simulink model "Arm_Simulation"  (R2022b)
settings: Solver=ode23t  StartTime=0.0  StopTime=10  RelTol=1e-3
undefined symbols (not defined in the file or in its folder): alpha, LF, Ts, X, Y, Z
libraries: sm_lib x16, nesl_utility x8, spsEdgeDetectorLib x6, instrumentseriallib x3, simulink_extras x3, simulink x2, svdutilitieslib x1
(part 1 of 2)
settings Model: PacingRate=10  Creator=gotta  LastModifiedBy=gotta
settings ExplorerConfigSet: InternalSimMechanicsExplorerSettings="<ExplorerConfiguration><canonicalview>default</canonicalview><AnimationSetting><BasePlaybackSpeed>1.0</BasePlaybackSpeed><PlaybackSpeedFactor>1.0</PlaybackSpeedFactor></AnimationSetting><TilePanel><TileInfo><Tiles Columns=\"2\" Count=\"3\" Rows=\"2\"><Column Weight=\"0.4994\"/><Column Weight=\"0.5006\"/><Row Weight=\"0.4993\"/><Row Weight=\"0.5007\"/><Tile Height=\"2\" Width=\"1\" X=\"0\" Y=\"0\"/><Tile Height=\"1\" Width=\"1\" X=\"1\" Y=\"0\"/><Tile Height=\"1\" Width=\"1\" X=\"1\" Y=\"1\"/></Tiles></TileInfo><SceneInfo><SceneViewer><BGColor><R>0.60000002384185791</R><G>0.60000002384185791</G><B>0.60000002384185791</B></BGColor><Camera><DoPerspective>off</DoPerspective><Position><X>0.130605904800483619</X><Y>-1.03965353021318974</Y><Z>0.165975841105155203</Z></Position><Center><X>0.130605904800483619</X><Y>-0.039653530213189736</Y><Z>0.165975841105155203</Z></Center><Up><X>0</X><Y>-0</Y><Z>1</Z></Up><ViewLimDist>1</ViewLimDist><YLim>0.285256663070233507</YLim><XLim>0.289401740076538072</XLim></Camera></SceneViewer><SceneViewer><BGColor><R>0.60000002384185791</R><G>0.60000002384185791</G><B>0.60000002384185791</B></BGColor><Camera><DoPerspective>off</DoPerspective><Position><X>0.102066420747171926</X><Y>-0.000570082663057591005</Y><Z>1.10062331896404597</Z></Position><Center><X>0.102066420747171926</X><Y>-0.000570082663057591005</Y><Z>0.100623318964045971</Z></Center><Up><X>0</X><Y>1</Y><Z>-0</Z></Up><ViewLimDist>1</ViewLimDist><YLim>0.171233923815175632</YLim><XLim>0.352540431384185116</XLim></Camera></SceneViewer><SceneViewer><BGColor><R>0.60000002384185791</R><G>0.60000002384185791</G><B>0.60000002384185791</B></BGColor><Camera><DoPerspective>off</DoPerspective><Position><X>1.08629246460336626</X><Y>-0.00159593778916227759</Y><Z>0.183546684797173593</Z></Position><Center><X>0.086292464603366259</X><Y>-0.00159593778916227759</Y><Z>0.183546684797173593</Z></Center><Up><X>-0</X><Y>0</Y><Z>1</Z></Up><ViewLimDist>1</ViewLimDist><YLim>0.219665879586588786</YLim><XLim>0.452253281501800386</XLim></Camera></SceneViewer></SceneInfo></TilePanel><MechEditorPanel><Cameras/><GfxPanelCameraMap/><VideoCreator><PlaybackSpeedRatio>1.0</PlaybackSpeedRatio><FrameRate>30</FrameRate><VideoFormat>Motion JPEG AVI</VideoFormat><FrameSize>auto</FrameSize></VideoCreator></MechEditorPanel></ExplorerConfiguration>"

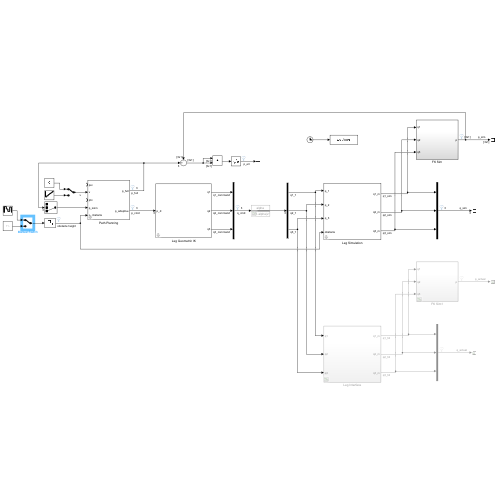
[thumbnail: Simulink's stored preview of the top-level diagram]
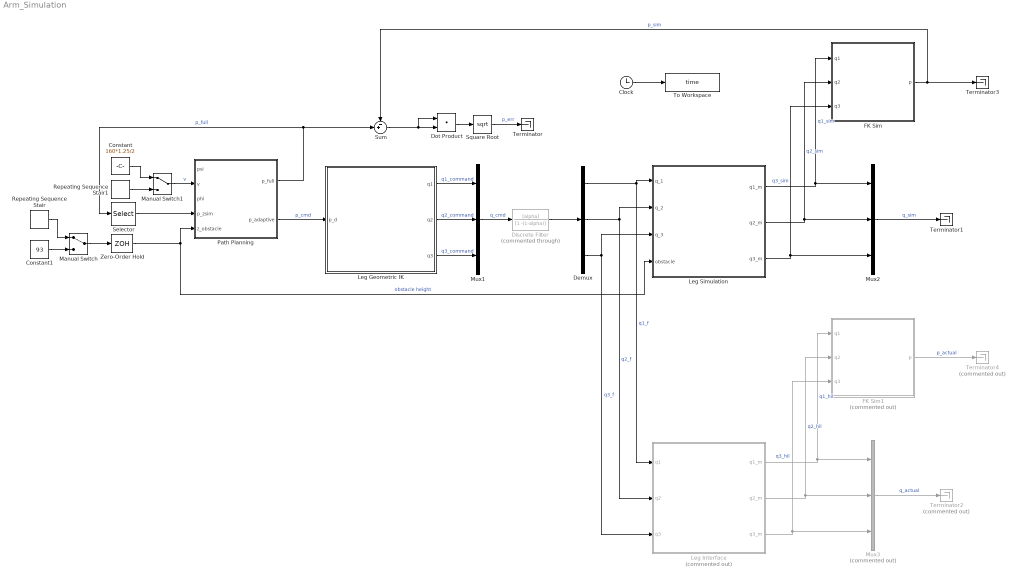
== system Arm_Simulation ==
  " Leg Geometric IK" : Subsystem  mask{coxa_length=40, femur_length=78, tibia_length=132, offset=178}
      mask prompts: coxa_length "Coxa Length [mm]:"; femur_length "Femur Length [mm]:"; tibia_length "Tibia Length [mm]:"; offset "Offset [mm]:"
  Clock : Clock
  Constant : Constant  Value=160*1.25/2
  Constant1 : Constant  Value=93
  Demux : Demux  Outputs=3
  Discrete Filter : DiscreteFilter  Commented=through  Numerator=[alpha]  Denominator=[1 -(1-alpha)]  SampleTime=Ts
  Dot Product : DotProduct  OutDataTypeStr=Inherit: Inherit via internal rule
  FK Sim : Subsystem
  FK Sim1 : Subsystem  Commented=on
  Leg Interface : Subsystem  Commented=on
  Leg Simulation : Subsystem  mask{RotationAngle=0.0}
      mask prompts: RotationAngle "Angular Offset [deg]:"
      mask TypeOptions RotationAngle: rotation/RotationAngle
  Manual Switch : ManualSwitch
  Manual Switch1 : ManualSwitch
  Mux1 : Mux  Inputs=3
  Mux2 : Mux  Inputs=3
  Mux3 : Mux  Commented=on  Inputs=3
  Path Planning : Subsystem  mask{Cx=155, Cy=0, Cz=93, r_o=60, n=1000, beta=0.6}
      mask prompts: Cx "X"; Cy "Y"; Cz "Z"; r_o "OWR Radius [mm]:"; n "Samples per Cycle:"; beta "Duty Factor beta:"
      mask DialogControl ParameterGroupVar Prompt: Rest Position [mm]
  Repeating Sequence Stair : simulink/Sources/Repeating Sequence Stair  OutValues=[93, 140, 140, 120, 120, 100, 100, 135, 135, 93]  tsamp=1  OutMin=[]  OutMax=[]  OutDataTypeStr=double  OutputDataTypeScalingMode=double  OutDataType=fixdt(0,8)  ConRadixGroup=Best Precision: Vector-wise  OutScaling=2^-12
  Repeating Sequence Stair1 : simulink/Sources/Repeating Sequence Stair  OutValues=[67:67/5:134]  tsamp=5  OutMin=[]  OutMax=[]  OutDataTypeStr=double  OutputDataTypeScalingMode=double  OutDataType=fixdt(0,8)  ConRadixGroup=Best Precision: Vector-wise  OutScaling=2^-12
  Selector : Selector  InputPortWidth=3  IndexOptions=Index vector (dialog)  Indices=3  OutputSizes=1
  Square Root : Sqrt
  Sum : Sum  Inputs=-+|
  Terminator : Terminator
  Terminator1 : Terminator
  Terminator2 : Terminator  Commented=on
  Terminator3 : Terminator
  Terminator4 : Terminator  Commented=on
  To Workspace : ToWorkspace  VariableName=time  SampleTime=1e-4
      settings: Save2DSignal=2-D array (concatenate along first dimension)
  Zero-Order Hold : ZeroOrderHold  SampleTime=1e-3
  wires:
  Leg Interface/3(q3_m) -> FK Sim1/3(q3), Mux3/3  "q3_hil"
  Leg Interface/2(q2_m) -> FK Sim1/2(q2), Mux3/2  "q2_hil"
  Leg Interface/1(q1_m) -> FK Sim1/1(q1), Mux3/1  "q1_hil"
  Leg Simulation/3(q3_m) -> Mux2/3, FK Sim/3(q3)  "q3_sim"
  Leg Simulation/2(q2_m) -> Mux2/2, FK Sim/2(q2)  "q2_sim"
  Leg Simulation/1(q1_m) -> Mux2/1, FK Sim/1(q1)  "q1_sim"
  Path Planning/1(p_full) -> Sum/2, Selector/1  "p_full"
  FK Sim/1(p) -> Terminator3/1, Sum/1  "p_sim"
  " Leg Geometric IK"/3(q3) -> Mux1/3  "q3_command"
  " Leg Geometric IK"/2(q2) -> Mux1/2  "q2_command"
  " Leg Geometric IK"/1(q1) -> Mux1/1  "q1_command"
  Demux/1 -> Leg Interface/1(q1), Leg Simulation/1(q_1)  "q1_f"
  Demux/2 -> Leg Interface/2(q2), Leg Simulation/2(q_2)  "q2_f"
  Demux/3 -> Leg Interface/3(q3), Leg Simulation/3(q_3)  "q3_f"
  Mux1/1 -> Discrete Filter/1  "q_cmd"
  Discrete Filter/1 -> Demux/1
  Constant/1 -> Manual Switch1/1
  Mux2/1 -> Terminator1/1  "q_sim"
  Mux3/1 -> Terminator2/1  "q_actual"
  FK Sim1/1(p) -> Terminator4/1  "p_actual"
  Selector/1 -> Path Planning/4(p_zsim)
  Repeating Sequence Stair1/1 -> Manual Switch1/2
  Manual Switch1/1 -> Path Planning/2(v)  "v"
  Clock/1 -> To Workspace/1
  Sum/1 -> Dot Product/1, Dot Product/2
  Dot Product/1 -> Square Root/1
  Square Root/1 -> Terminator/1  "p_err"
  Repeating Sequence Stair/1 -> Manual Switch/1
  Zero-Order Hold/1 -> Leg Simulation/4(obstacle), Path Planning/5(z_obstacle)  "obstacle height"
  Path Planning/2(p_adaptive) -> " Leg Geometric IK"/1(p_d)  "p_cmd"
  Constant1/1 -> Manual Switch/2
  Manual Switch/1 -> Zero-Order Hold/1

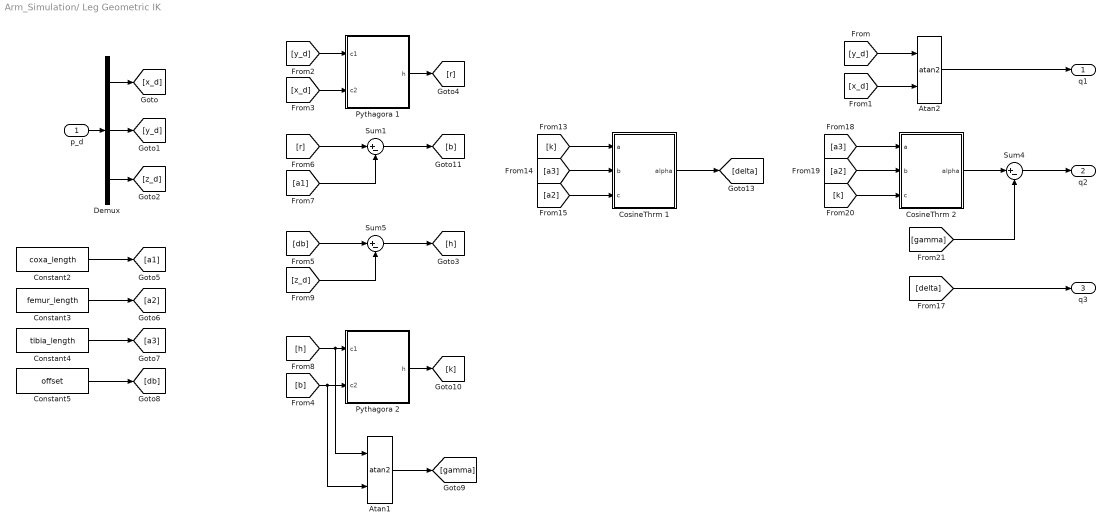
== system Arm_Simulation/ Leg Geometric IK ==
  p_d : Inport
  Atan1 : Trigonometry  Operator=atan2
  Atan2 : Trigonometry  Operator=atan2
  Constant2 : Constant  Value=coxa_length
  Constant3 : Constant  Value=femur_length
  Constant4 : Constant  Value=tibia_length
  Constant5 : Constant  Value=offset
  CosineThrm 1 : Subsystem
  CosineThrm 2 : Subsystem
  Demux : Demux  Outputs=3
  Pythagora 1 : Subsystem
  Pythagora 2 : Subsystem
  Sum1 : Sum  Inputs=|+-
  Sum4 : Sum  Inputs=|+-
  Sum5 : Sum  Inputs=|+-
  q1 : Outport
  q2 : Outport  Port=2
  q3 : Outport  Port=3
  wires:
  p_d/1 -> Demux/1
  Demux/3 -> [z_d]
  Atan2/1 -> q1/1
  Demux/1 -> [x_d]
  Demux/2 -> [y_d]
  [y_d] -> Atan2/1
  [x_d] -> Atan2/2
  Pythagora 1/1(h) -> [r]
  [y_d] -> Pythagora 1/1(c1)
  [x_d] -> Pythagora 1/2(c2)
  Constant4/1 -> [a3]
  Constant3/1 -> [a2]
  Constant2/1 -> [a1]
  [a1] -> Sum1/2
  [r] -> Sum1/1
  Sum1/1 -> [b]
  [b] -> Atan1/2, Pythagora 2/2(c2)
  [h] -> Atan1/1, Pythagora 2/1(c1)
  Pythagora 2/1(h) -> [k]
  CosineThrm 1/1(alpha) -> [delta]
  [a2] -> CosineThrm 1/3(c)
  [a3] -> CosineThrm 1/2(b)
  [k] -> CosineThrm 1/1(a)
  [a3] -> CosineThrm 2/1(a)
  [a2] -> CosineThrm 2/2(b)
  [k] -> CosineThrm 2/3(c)
  CosineThrm 2/1(alpha) -> Sum4/1
  Sum4/1 -> q2/1
  [gamma] -> Sum4/2
  Sum5/1 -> [h]
  [db] -> Sum5/1
  [z_d] -> Sum5/2
  Constant5/1 -> [db]
  Atan1/1 -> [gamma]
  [delta] -> q3/1

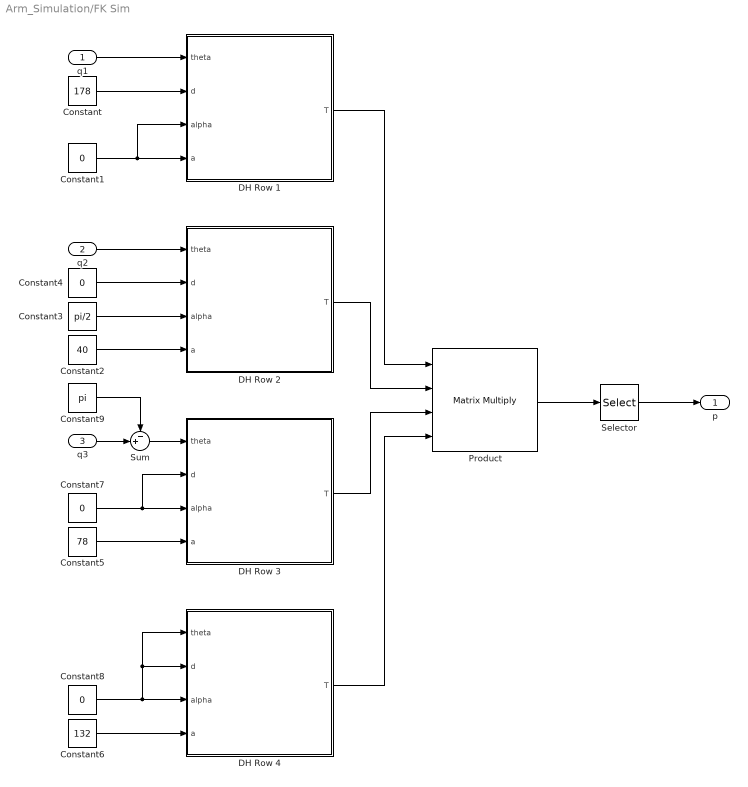
== system Arm_Simulation/FK Sim ==
  q1 : Inport
  q2 : Inport  Port=2
  q3 : Inport  Port=3
  Constant : Constant  Value=178
  Constant{1,4,7..8} (4 alike) : Constant  Value=0
  Constant2 : Constant  Value=40
  Constant3 : Constant  Value=pi/2
  Constant5 : Constant  Value=78
  Constant6 : Constant  Value=132
  Constant9 : Constant  Value=pi
  DH Row 1 : MATLAB Function  TreatAsAtomicUnit=on
  DH Row 2 : MATLAB Function  TreatAsAtomicUnit=on
  DH Row 3 : MATLAB Function  TreatAsAtomicUnit=on
  DH Row 4 : MATLAB Function  TreatAsAtomicUnit=on
  Product : Product  Inputs=4  Multiplication=Matrix(*)
  Selector : Selector  NumberOfDimensions=2  InputPortWidth=3  IndexOptions=Index vector (dialog),Index vector (dialog)  Indices=[1 2 3],4  OutputSizes=1,1
  Sum : Sum  Inputs=-+|
  p : Outport
  wires:
  q1/1 -> DH Row 1/1(theta)
  Constant/1 -> DH Row 1/2(d)
  Constant1/1 -> DH Row 1/3(alpha), DH Row 1/4(a)
  q2/1 -> DH Row 2/1(theta)
  Constant4/1 -> DH Row 2/2(d)
  Constant3/1 -> DH Row 2/3(alpha)
  Constant2/1 -> DH Row 2/4(a)
  Constant5/1 -> DH Row 3/4(a)
  Constant7/1 -> DH Row 3/3(alpha), DH Row 3/2(d)
  q3/1 -> Sum/2
  Constant8/1 -> DH Row 4/3(alpha), DH Row 4/1(theta), DH Row 4/2(d)
  Constant6/1 -> DH Row 4/4(a)
  DH Row 1/1(T) -> Product/1
  DH Row 2/1(T) -> Product/2
  DH Row 3/1(T) -> Product/3
  DH Row 4/1(T) -> Product/4
  Product/1 -> Selector/1
  Selector/1 -> p/1
  Sum/1 -> DH Row 3/1(theta)
  Constant9/1 -> Sum/1

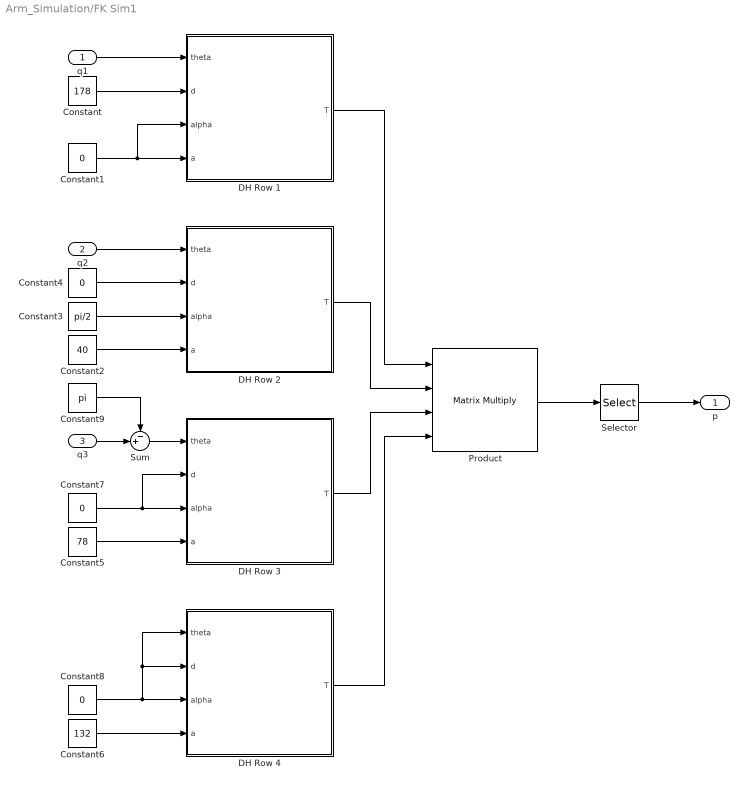
== system Arm_Simulation/FK Sim1 ==
  q1 : Inport
  q2 : Inport  Port=2
  q3 : Inport  Port=3
  Constant : Constant  Value=178
  Constant{1,4,7..8} (4 alike) : Constant  Value=0
  Constant2 : Constant  Value=40
  Constant3 : Constant  Value=pi/2
  Constant5 : Constant  Value=78
  Constant6 : Constant  Value=132
  Constant9 : Constant  Value=pi
  DH Row 1 : MATLAB Function  TreatAsAtomicUnit=on
  DH Row 2 : MATLAB Function  TreatAsAtomicUnit=on
  DH Row 3 : MATLAB Function  TreatAsAtomicUnit=on
  DH Row 4 : MATLAB Function  TreatAsAtomicUnit=on
  Product : Product  Inputs=4  Multiplication=Matrix(*)
  Selector : Selector  NumberOfDimensions=2  InputPortWidth=3  IndexOptions=Index vector (dialog),Index vector (dialog)  Indices=[1 2 3],4  OutputSizes=1,1
  Sum : Sum  Inputs=-+|
  p : Outport
  wires:
  Constant9/1 -> Sum/1
  Sum/1 -> DH Row 3/1(theta)
  Selector/1 -> p/1
  Product/1 -> Selector/1
  DH Row 4/1(T) -> Product/4
  DH Row 3/1(T) -> Product/3
  DH Row 2/1(T) -> Product/2
  DH Row 1/1(T) -> Product/1
  Constant6/1 -> DH Row 4/4(a)
  Constant8/1 -> DH Row 4/2(d), DH Row 4/1(theta), DH Row 4/3(alpha)
  q3/1 -> Sum/2
  Constant7/1 -> DH Row 3/2(d), DH Row 3/3(alpha)
  Constant5/1 -> DH Row 3/4(a)
  Constant2/1 -> DH Row 2/4(a)
  Constant3/1 -> DH Row 2/3(alpha)
  Constant4/1 -> DH Row 2/2(d)
  q2/1 -> DH Row 2/1(theta)
  Constant1/1 -> DH Row 1/4(a), DH Row 1/3(alpha)
  Constant/1 -> DH Row 1/2(d)
  q1/1 -> DH Row 1/1(theta)

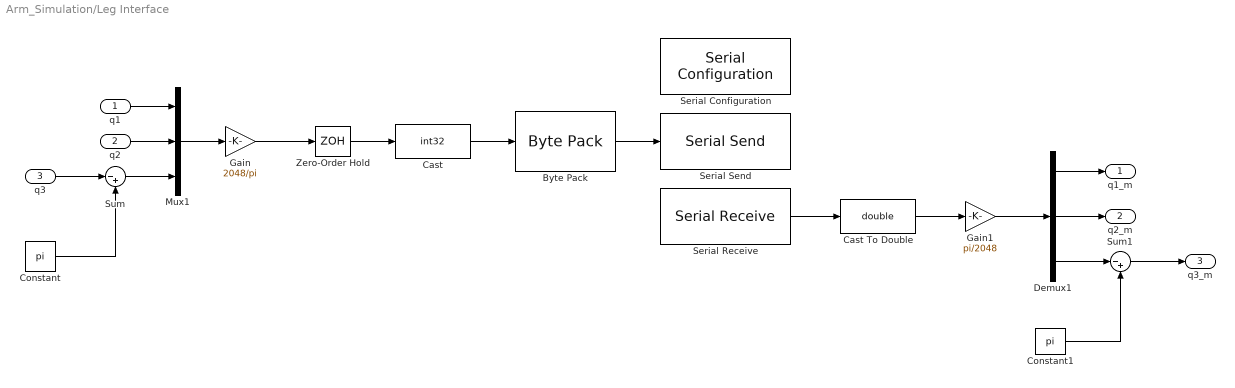
== system Arm_Simulation/Leg Interface ==
  q1 : Inport
  q2 : Inport  Port=2
  q3 : Inport  Port=3
  Byte Pack : svdutilitieslib/Byte Pack  maskPackedDataType=uint8  datatypes={'int32'}  byteAlign=1  blockPlatform=arduinoert
  Cast : DataTypeConversion  OutDataTypeStr=int32  SaturateOnIntegerOverflow=off  RndMeth=Floor
  Cast To Double : DataTypeConversion  OutDataTypeStr=double  SaturateOnIntegerOverflow=off  RndMeth=Floor
  Constant : Constant  Value=pi
  Constant1 : Constant  Value=pi
  Demux1 : Demux  Outputs=3
  Gain : Gain  Gain=2048/pi
  Gain1 : Gain  Gain=pi/2048
  Mux1 : Mux  Inputs=3
  Serial Configuration : instrumentseriallib/Serial Configuration  Priority=-200000  PortSel=COM6  Port=COM6  ComPort=COM6  BaudRate=115200  DataBits=8  Parity=none  StopBits=1  ByteOrder=little-endian  FlowControl=none  Timeout=10  SimulateUsing=Interpreted execution  BlockInModel=on  aMode=1
  Serial Receive : instrumentseriallib/Serial Receive  Priority=1  PortSel=COM6  Port=COM6  ComPort=COM6  DataType=int32  SaveDataType=uint8  ToggleHeader=on  Header='A'  ToggleTerminator=on  Terminator=LF ('\n')  CustomTerminator=[]  InputFormat=Column major  ToggleDataSize=on  DataSize=[1 3]  EnableBlockingMode=on  ActionDataUnavailable=Output last received value  ActionWhenDataUnavailable=Output last received value  CustomValue=0  SampleTime=1e-2  SimulateUsing=Interpreted execution  BlockInModel=on  aMode=1
  Serial Send : instrumentseriallib/Serial Send  Priority=1  PortSel=COM6  Port=COM6  ComPort=COM6  Header=[]  Terminator=<none>  CustomTerminator=[]  EnableBlockingMode=on  SimulateUsing=Interpreted execution  BlockInModel=on  aMode=1
  Sum : Sum  Inputs=|-+
  Sum1 : Sum  Inputs=|-+
  Zero-Order Hold : ZeroOrderHold  SampleTime=1e-2
  q1_m : Outport
  q2_m : Outport  Port=2
  q3_m : Outport  Port=3
  wires:
  Cast/1 -> Byte Pack/1
  Serial Receive/1 -> Cast To Double/1
  Mux1/1 -> Gain/1
  Demux1/2 -> q2_m/1
  Demux1/1 -> q1_m/1
  q1/1 -> Mux1/1
  q2/1 -> Mux1/2
  Cast To Double/1 -> Gain1/1
  Gain1/1 -> Demux1/1
  Gain/1 -> Zero-Order Hold/1
  Byte Pack/1 -> Serial Send/1
  Zero-Order Hold/1 -> Cast/1
  Sum/1 -> Mux1/3
  q3/1 -> Sum/1
  Constant/1 -> Sum/2
  Constant1/1 -> Sum1/2
  Sum1/1 -> q3_m/1
  Demux1/3 -> Sum1/1

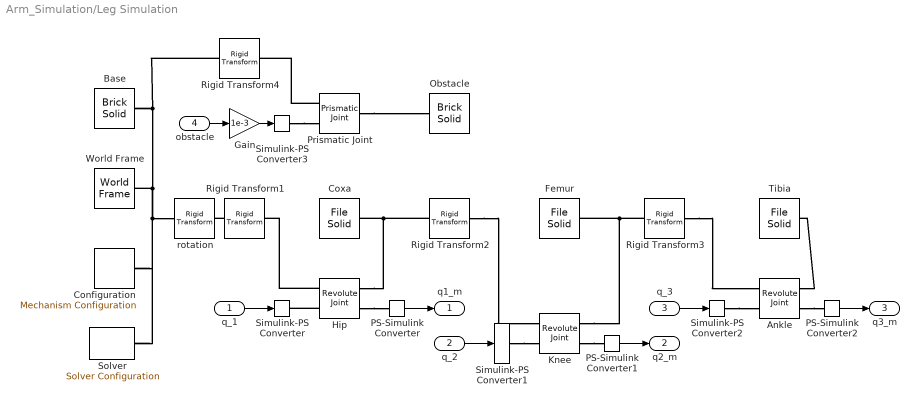
== system Arm_Simulation/Leg Simulation ==
  q_1 : Inport
  q_2 : Inport  Port=2
  q_3 : Inport  Port=3
  obstacle : Inport  Port=4
  Ankle : sm_lib/Joints/Revolute Joint  JointMode=Normal  SenseConstraintForce=off  SenseConstraintForceX=off  SenseConstraintForceY=off  SenseConstraintForceZ=off  SenseConstraintTorque=off  SenseConstraintTorqueX=off  SenseConstraintTorqueY=off  SenseConstraintTorqueZ=off  SenseTotalForce=off  SenseTotalForceX=off  SenseTotalForceY=off  SenseTotalForceZ=off  SenseTotalTorque=off  SenseTotalTorqueX=off  SenseTotalTorqueY=off  SenseTotalTorqueZ=off  CompositeWrenchDir=FollowerOnBase  CompositeWrenchFrame=BaseFrame  EquilibriumPosition=0  EquilibriumPositionUnits=deg  SpringStiffness=0  SpringStiffnessUnits=N*m/deg  DampingCoefficient=0  DampingCoefficientUnits=N*m/(deg/s)  TorqueActuationMode=ComputedTorque  MotionActuationMode=InputMotion  SensePosition=on  SenseVelocity=off  SenseAcceleration=off  SenseTorqueForce=off  SenseLowerLimitTorqueForce=off  SenseUpperLimitTorqueForce=off  LowerLimitSpecify=off  LowerLimitBound=-90  LowerLimitBoundUnits=deg  LowerLimitStiffness=1e4  LowerLimitStiffnessUnits=N*m/deg  LowerLimitDamping=10  LowerLimitDampingUnits=N*m/(deg/s)  LowerLimitTransitionRegionWidth=0.1  LowerLimitTransitionRegionWidthUnits=deg  UpperLimitSpecify=off  UpperLimitBound=90  UpperLimitBoundUnits=deg  UpperLimitStiffness=1e4  UpperLimitStiffnessUnits=N*m/deg  UpperLimitDamping=10  UpperLimitDampingUnits=N*m/(deg/s)  UpperLimitTransitionRegionWidth=0.1  UpperLimitTransitionRegionWidthUnits=deg  PositionTargetSpecify=off  PositionTargetPriority=High  PositionTargetValue=0  PositionTargetValueUnits=deg  VelocityTargetSpecify=off  VelocityTargetPriority=High  VelocityTargetValue=0  VelocityTargetValueUnits=deg/s
  Base : sm_lib/Body Elements/Brick Solid  GraphicAmbientColor=[0.15 0.15 0.15 1.0]  BasedOnType=Density  BrickDimensions=[15 15 200]  BrickDimensionUnits=mm  CenterOfMass=[0 0 0]  CenterOfMassUnits=m  GraphicDiffuseColor=[0.0 0.0 0.0]  Density=1000  DensityUnits=kg/m^3  DoExposeReferenceFrame=on  GraphicEmissiveColor=[0.0 0.0 0.0 1.0]  ExportEntireGeometry=off  SerializedFrames=<Frames><Frame><Id>Frame1</Id><Value><Name>Fb</Name><Origin><Source>GeometricFeature</Source><FeatureName>-z surface</FeatureName></Origin><PrimaryAxis><DefinedDirection>+Z</DefinedDirection><Source>CenterOfMassFrame</Source><SourceDirection>+Z</SourceDirection><FeatureName></FeatureName></PrimaryAxis><SecondaryAxis><DefinedDirection>+X</DefinedDirection><Source>GeometricFeature</Source><SourceDirection>+X</SourceDirection><FeatureName>-y -z curve</FeatureName></SecondaryAxis></Value></Frame></Frames>  MarkerShape=Sphere  MarkerSize=10  GraphicType=FromGeometry  InertiaType=CalculateFromGeometry  Mass=1  MassUnits=kg  MomentsOfInertia=[1 1 1]  MomentsOfInertiaUnits=kg*m^2  GraphicOpacity=1.0  ProductsOfInertia=[0 0 0]  ProductsOfInertiaUnits=kg*m^2  GraphicShininess=75  GraphicSpecularColor=[0.5 0.5 0.5 1.0]  GraphicVisPropType=SimpleVisualProperties
  Configuration : sm_lib/Utilities/Mechanism Configuration  UniformGravity=Constant  GravityVector=[0 0 -9.80665]  GravityUnits=m/s^2  LinearizationDelta=0.001  JointModeTransitionNonlinearIterations=2
  Coxa : sm_lib/Body Elements/File Solid  ExtGeomFileName=D:\Data\_PROGETTI\PRJ_SMART_SERVO\MATLAB\Arm Simulation\3D Models\coxa.stl  UnitType=Custom  ExtGeomFileUnits=mm  StepReaderType=HEX  ExportConvexHullGeometry=off  InertiaType=CalculateFromGeometry  Mass=1  MassUnits=kg  CenterOfMass=[0 0 0]  CenterOfMassUnits=m  MomentsOfInertia=[1 1 1]  MomentsOfInertiaUnits=kg*m^2  ProductsOfInertia=[0 0 0]  ProductsOfInertiaUnits=kg*m^2  BasedOnType=Density  Density=1200  DensityUnits=kg/m^3  DoExposeReferenceFrame=on  SerializedFrames=<Frames><Frame><Id>Frame1</Id><Value><Name>F1</Name><Origin><Source>ReferenceFrame</Source><FeatureName></FeatureName></Origin><PrimaryAxis><DefinedDirection>+Z</DefinedDirection><Source>ReferenceFrame</Source><SourceDirection>-Z</SourceDirection><FeatureName></FeatureName></PrimaryAxis><SecondaryAxis><DefinedDirection>+X</DefinedDirection><Source>ReferenceFrame</Source><SourceDirection>+X</SourceDirection><FeatureName></FeatureName></SecondaryAxis></Value></Frame></Frames>  GraphicType=FromGeometry  MarkerShape=Sphere  MarkerSize=10  GraphicVisPropType=SimpleVisualProperties  GraphicDiffuseColor=[1.0 0.2 0.2]  GraphicSpecularColor=[0.5 0.5 0.5 1.0]  GraphicAmbientColor=[0.15 0.15 0.15 1.0]  GraphicEmissiveColor=[0.0 0.0 0.0 1.0]  GraphicShininess=75  GraphicOpacity=1.0
  Femur : sm_lib/Body Elements/File Solid  ExtGeomFileName=D:\Data\_PROGETTI\PRJ_SMART_SERVO\MATLAB\Arm Simulation\3D Models\femur.stl  UnitType=Custom  ExtGeomFileUnits=mm  StepReaderType=HEX  ExportConvexHullGeometry=off  InertiaType=CalculateFromGeometry  Mass=1  MassUnits=kg  CenterOfMass=[0 0 0]  CenterOfMassUnits=m  MomentsOfInertia=[1 1 1]  MomentsOfInertiaUnits=kg*m^2  ProductsOfInertia=[0 0 0]  ProductsOfInertiaUnits=kg*m^2  BasedOnType=Density  Density=1200  DensityUnits=kg/m^3  DoExposeReferenceFrame=on  SerializedFrames=<Frames/>  GraphicType=FromGeometry  MarkerShape=Sphere  MarkerSize=10  GraphicVisPropType=SimpleVisualProperties  GraphicDiffuseColor=[0.6 0.8 0.0]  GraphicSpecularColor=[0.5 0.5 0.5 1.0]  GraphicAmbientColor=[0.15 0.15 0.15 1.0]  GraphicEmissiveColor=[0.0 0.0 0.0 1.0]  GraphicShininess=75  GraphicOpacity=1.0
  Gain : Gain  Gain=1e-3
  Hip : sm_lib/Joints/Revolute Joint  JointMode=Normal  SenseConstraintForce=off  SenseConstraintForceX=off  SenseConstraintForceY=off  SenseConstraintForceZ=off  SenseConstraintTorque=off  SenseConstraintTorqueX=off  SenseConstraintTorqueY=off  SenseConstraintTorqueZ=off  SenseTotalForce=off  SenseTotalForceX=off  SenseTotalForceY=off  SenseTotalForceZ=off  SenseTotalTorque=off  SenseTotalTorqueX=off  SenseTotalTorqueY=off  SenseTotalTorqueZ=off  CompositeWrenchDir=FollowerOnBase  CompositeWrenchFrame=BaseFrame  EquilibriumPosition=0  EquilibriumPositionUnits=deg  SpringStiffness=0  SpringStiffnessUnits=N*m/deg  DampingCoefficient=0  DampingCoefficientUnits=N*m/(deg/s)  TorqueActuationMode=ComputedTorque  MotionActuationMode=InputMotion  SensePosition=on  SenseVelocity=off  SenseAcceleration=off  SenseTorqueForce=off  SenseLowerLimitTorqueForce=off  SenseUpperLimitTorqueForce=off  LowerLimitSpecify=off  LowerLimitBound=-90  LowerLimitBoundUnits=deg  LowerLimitStiffness=1e4  LowerLimitStiffnessUnits=N*m/deg  LowerLimitDamping=10  LowerLimitDampingUnits=N*m/(deg/s)  LowerLimitTransitionRegionWidth=0.1  LowerLimitTransitionRegionWidthUnits=deg  UpperLimitSpecify=off  UpperLimitBound=90  UpperLimitBoundUnits=deg  UpperLimitStiffness=1e4  UpperLimitStiffnessUnits=N*m/deg  UpperLimitDamping=10  UpperLimitDampingUnits=N*m/(deg/s)  UpperLimitTransitionRegionWidth=0.1  UpperLimitTransitionRegionWidthUnits=deg  PositionTargetSpecify=off  PositionTargetPriority=High  PositionTargetValue=0  PositionTargetValueUnits=deg  VelocityTargetSpecify=off  VelocityTargetPriority=High  VelocityTargetValue=0  VelocityTargetValueUnits=deg/s
  Knee : sm_lib/Joints/Revolute Joint  JointMode=Normal  SenseConstraintForce=off  SenseConstraintForceX=off  SenseConstraintForceY=off  SenseConstraintForceZ=off  SenseConstraintTorque=off  SenseConstraintTorqueX=off  SenseConstraintTorqueY=off  SenseConstraintTorqueZ=off  SenseTotalForce=off  SenseTotalForceX=off  SenseTotalForceY=off  SenseTotalForceZ=off  SenseTotalTorque=off  SenseTotalTorqueX=off  SenseTotalTorqueY=off  SenseTotalTorqueZ=off  CompositeWrenchDir=FollowerOnBase  CompositeWrenchFrame=BaseFrame  EquilibriumPosition=0  EquilibriumPositionUnits=deg  SpringStiffness=0  SpringStiffnessUnits=N*m/deg  DampingCoefficient=0  DampingCoefficientUnits=N*m/(deg/s)  TorqueActuationMode=ComputedTorque  MotionActuationMode=InputMotion  SensePosition=on  SenseVelocity=off  SenseAcceleration=off  SenseTorqueForce=off  SenseLowerLimitTorqueForce=off  SenseUpperLimitTorqueForce=off  LowerLimitSpecify=off  LowerLimitBound=-90  LowerLimitBoundUnits=deg  LowerLimitStiffness=1e4  LowerLimitStiffnessUnits=N*m/deg  LowerLimitDamping=10  LowerLimitDampingUnits=N*m/(deg/s)  LowerLimitTransitionRegionWidth=0.1  LowerLimitTransitionRegionWidthUnits=deg  UpperLimitSpecify=off  UpperLimitBound=90  UpperLimitBoundUnits=deg  UpperLimitStiffness=1e4  UpperLimitStiffnessUnits=N*m/deg  UpperLimitDamping=10  UpperLimitDampingUnits=N*m/(deg/s)  UpperLimitTransitionRegionWidth=0.1  UpperLimitTransitionRegionWidthUnits=deg  PositionTargetSpecify=off  PositionTargetPriority=High  PositionTargetValue=0  PositionTargetValueUnits=deg  VelocityTargetSpecify=off  VelocityTargetPriority=High  VelocityTargetValue=0  VelocityTargetValueUnits=deg/s
  Obstacle : sm_lib/Body Elements/Brick Solid  GraphicAmbientColor=[0.15 0.15 0.15 1.0]  BasedOnType=Density  BrickDimensions=[100 200 10]  BrickDimensionUnits=mm  CenterOfMass=[0 0 0]  CenterOfMassUnits=m  GraphicDiffuseColor=[0.2 0.6 1.0]  Density=1000  DensityUnits=kg/m^3  DoExposeReferenceFrame=on  GraphicEmissiveColor=[0.0 0.0 0.0 1.0]  ExportEntireGeometry=off  SerializedFrames=<Frames/>  MarkerShape=Sphere  MarkerSize=10  GraphicType=FromGeometry  InertiaType=CalculateFromGeometry  Mass=1  MassUnits=kg  MomentsOfInertia=[1 1 1]  MomentsOfInertiaUnits=kg*m^2  GraphicOpacity=1.0  ProductsOfInertia=[0 0 0]  ProductsOfInertiaUnits=kg*m^2  GraphicShininess=75  GraphicSpecularColor=[0.5 0.5 0.5 1.0]  GraphicVisPropType=SimpleVisualProperties
  PS-Simulink Converter : nesl_utility/PS-Simulink Converter  PhysicalDomain=network_engine_domain  SubClassName=ps_output  LeftPortType=input  RightPortType=output  PseudoPeriodic=off  Frequencies=[]  VectorFormat=inherit  Unit=inherit  AffineConversion=off
  PS-Simulink Converter1 : nesl_utility/PS-Simulink Converter  PhysicalDomain=network_engine_domain  SubClassName=ps_output  LeftPortType=input  RightPortType=output  PseudoPeriodic=off  Frequencies=[]  VectorFormat=inherit  Unit=inherit  AffineConversion=off
  PS-Simulink Converter2 : nesl_utility/PS-Simulink Converter  PhysicalDomain=network_engine_domain  SubClassName=ps_output  LeftPortType=input  RightPortType=output  PseudoPeriodic=off  Frequencies=[]  VectorFormat=inherit  Unit=inherit  AffineConversion=off
  Prismatic Joint : sm_lib/Joints/Prismatic Joint  JointMode=Normal  SenseConstraintForce=off  SenseConstraintForceX=off  SenseConstraintForceY=off  SenseConstraintForceZ=off  SenseConstraintTorque=off  SenseConstraintTorqueX=off  SenseConstraintTorqueY=off  SenseConstraintTorqueZ=off  SenseTotalForce=off  SenseTotalForceX=off  SenseTotalForceY=off  SenseTotalForceZ=off  SenseTotalTorque=off  SenseTotalTorqueX=off  SenseTotalTorqueY=off  SenseTotalTorqueZ=off  CompositeWrenchDir=FollowerOnBase  CompositeWrenchFrame=BaseFrame  EquilibriumPosition=0  EquilibriumPositionUnits=m  SpringStiffness=0  SpringStiffnessUnits=N/m  DampingCoefficient=0  DampingCoefficientUnits=N/(m/s)  TorqueActuationMode=ComputedTorque  MotionActuationMode=InputMotion  SensePosition=off  SenseVelocity=off  SenseAcceleration=off  SenseTorqueForce=off  SenseLowerLimitTorqueForce=off  SenseUpperLimitTorqueForce=off  LowerLimitSpecify=off  LowerLimitBound=-1  LowerLimitBoundUnits=m  LowerLimitStiffness=1e6  LowerLimitStiffnessUnits=N/m  LowerLimitDamping=1e3  LowerLimitDampingUnits=N/(m/s)  LowerLimitTransitionRegionWidth=1e-4  LowerLimitTransitionRegionWidthUnits=m  UpperLimitSpecify=off  UpperLimitBound=1  UpperLimitBoundUnits=m  UpperLimitStiffness=1e6  UpperLimitStiffnessUnits=N/m  UpperLimitDamping=1e3  UpperLimitDampingUnits=N/(m/s)  UpperLimitTransitionRegionWidth=1e-4  UpperLimitTransitionRegionWidthUnits=m  PositionTargetSpecify=off  PositionTargetPriority=High  PositionTargetValue=0  PositionTargetValueUnits=m  VelocityTargetSpecify=off  VelocityTargetPriority=High  VelocityTargetValue=0  VelocityTargetValueUnits=m/s
  Rigid Transform1 : sm_lib/Frames and Transforms/Rigid Transform  TranslationMethod=Cartesian  TranslationStandardOffset=100  TranslationLengthUnit=mm  TranslationStandardAxis=+Z  TranslationCartesianOffset=[50 0 178]  TranslationROffset=0  TranslationROffsetUnits=m  TranslationZOffset=0  TranslationZOffsetUnits=m  TranslationThetaOffset=0  TranslationThetaOffsetUnits=deg  RotationMethod=StandardAxis  RotationAngleUnits=deg  RotationStandardAxis=+Z  RotationAngle=0.0  RotationArbitraryAxis=[0 0 1]  FollAlignAxisA=+X  BaseAlignAxisA=+Y  FollAlignAxisB=+Y  BaseAlignAxisB=+Z  RotationSequenceAxes=FollowerAxes  RotationSequence=XYX  RotationSequenceAngles=[0 0 0]  RotationSequenceAnglesUnits=deg  RotationMatrix=[1 0 0; 0 1 0; 0 0 1]  Quaternion=[1 0 0 0]
  Rigid Transform2 : sm_lib/Frames and Transforms/Rigid Transform  TranslationMethod=StandardAxis  TranslationStandardOffset=40  TranslationLengthUnit=mm  TranslationStandardAxis=+X  TranslationCartesianOffset=[40 0 0]  TranslationROffset=0  TranslationROffsetUnits=m  TranslationZOffset=0  TranslationZOffsetUnits=m  TranslationThetaOffset=0  TranslationThetaOffsetUnits=deg  RotationMethod=StandardAxis  RotationAngleUnits=deg  RotationStandardAxis=+X  RotationAngle=90  RotationArbitraryAxis=[0 0 1]  FollAlignAxisA=+X  BaseAlignAxisA=+Y  FollAlignAxisB=+Y  BaseAlignAxisB=+Z  RotationSequenceAxes=FollowerAxes  RotationSequence=XYX  RotationSequenceAngles=[0 0 0]  RotationSequenceAnglesUnits=deg  RotationMatrix=[1 0 0; 0 1 0; 0 0 1]  Quaternion=[1 0 0 0]
  Rigid Transform3 : sm_lib/Frames and Transforms/Rigid Transform  TranslationMethod=StandardAxis  TranslationStandardOffset=78  TranslationLengthUnit=mm  TranslationStandardAxis=+X  TranslationCartesianOffset=[40 0 0]  TranslationROffset=0  TranslationROffsetUnits=m  TranslationZOffset=0  TranslationZOffsetUnits=m  TranslationThetaOffset=0  TranslationThetaOffsetUnits=deg  RotationMethod=None  RotationAngleUnits=deg  RotationStandardAxis=+X  RotationAngle=180  RotationArbitraryAxis=[0 0 1]  FollAlignAxisA=+X  BaseAlignAxisA=+Y  FollAlignAxisB=+Y  BaseAlignAxisB=+Z  RotationSequenceAxes=FollowerAxes  RotationSequence=XYX  RotationSequenceAngles=[0 0 0]  RotationSequenceAnglesUnits=deg  RotationMatrix=[1 0 0; 0 1 0; 0 0 1]  Quaternion=[1 0 0 0]
  Rigid Transform4 : sm_lib/Frames and Transforms/Rigid Transform  TranslationMethod=Cartesian  TranslationStandardOffset=100  TranslationLengthUnit=mm  TranslationStandardAxis=+Z  TranslationCartesianOffset=[205, 0, -5]  TranslationROffset=0  TranslationROffsetUnits=m  TranslationZOffset=0  TranslationZOffsetUnits=m  TranslationThetaOffset=0  TranslationThetaOffsetUnits=deg  RotationMethod=StandardAxis  RotationAngleUnits=deg  RotationStandardAxis=+Z  RotationAngle=0.0  RotationArbitraryAxis=[0 0 1]  FollAlignAxisA=+X  BaseAlignAxisA=+Y  FollAlignAxisB=+Y  BaseAlignAxisB=+Z  RotationSequenceAxes=FollowerAxes  RotationSequence=XYX  RotationSequenceAngles=[0 0 0]  RotationSequenceAnglesUnits=deg  RotationMatrix=[1 0 0; 0 1 0; 0 0 1]  Quaternion=[1 0 0 0]
  Simulink-PS Converter : nesl_utility/Simulink-PS Converter  PhysicalDomain=network_engine_domain  SubClassName=ps_input  LeftPortType=input  RightPortType=output  PseudoPeriodic=off  Frequencies=[]  NoiseDistribution=none  NoiseParameters=[]  Unit=1  AffineConversion=off  FilteringAndDerivatives=filter  SimscapeFilterOrder=2  InputFilterTimeConstant=0.001  UdotUserProvided=0
  Simulink-PS Converter1 : nesl_utility/Simulink-PS Converter  PhysicalDomain=network_engine_domain  SubClassName=ps_input  LeftPortType=input  RightPortType=output  PseudoPeriodic=off  Frequencies=[]  NoiseDistribution=none  NoiseParameters=[]  Unit=1  AffineConversion=off  FilteringAndDerivatives=filter  SimscapeFilterOrder=2  InputFilterTimeConstant=0.001  UdotUserProvided=1
  Simulink-PS Converter2 : nesl_utility/Simulink-PS Converter  PhysicalDomain=network_engine_domain  SubClassName=ps_input  LeftPortType=input  RightPortType=output  PseudoPeriodic=off  Frequencies=[]  NoiseDistribution=none  NoiseParameters=[]  Unit=1  AffineConversion=off  FilteringAndDerivatives=filter  SimscapeFilterOrder=2  InputFilterTimeConstant=0.001  UdotUserProvided=0
  Simulink-PS Converter3 : nesl_utility/Simulink-PS Converter  PhysicalDomain=network_engine_domain  SubClassName=ps_input  LeftPortType=input  RightPortType=output  PseudoPeriodic=off  Frequencies=[]  NoiseDistribution=none  NoiseParameters=[]  Unit=1  AffineConversion=off  FilteringAndDerivatives=filter  SimscapeFilterOrder=2  InputFilterTimeConstant=0.001  UdotUserProvided=0
  Solver : nesl_utility/Solver Configuration  PhysicalDomain=network_engine_domain  SubClassName=solver  LeftPortType=input  RightPortType=generic  Tones=[]  Harmonics=[]  SimulateNoise=off  Profile=off  UseLocalSampling=off  EnableSwitchedLinearOptims=on  FrequencyDomain=off  UseCCode=off  RelTol=0.001  AbsTol=0.001  MinStep=1e-09  ToWorkspace=off  RevertToSquareIcSolve=off  NumHomotopyIterations=100  PhasorMode=off  PhasorModeNumHarmonics=1  ConsistencySolver=NEWTON_XTOL_AFTER_FTOL  IndexReductionMethod=DerivativeReplacement  DoDC=off  ResidualTolerance=1e-09  ConsistencyTolSource=GLOBAL  ConsistencyAbsTol=0.001  ConsistencyRelTol=0.001  ConsistencyTolFactor=0.001  UseLocalSolver=off  LocalSolverChoice=NE_BACKWARD_EULER_ADVANCER  ResolveIndetEquations=on  FunctionEvalNumThread=1  LocalSolverSampleTime=0.001  DoFixedCost=off  MaxNonlinIter=3  MaxModeIter=2  ComputeImpulses=off  ImpulseIterations=2  LinearAlgebra=auto  LinearAlgebraNumThread=0  EquationFormulation=NE_TIME_EF  DelaysMemoryBudget=1024  AutomaticFiltering=on  FilteringTimeConstant=0.001  PartitionStorageMethod=AS_NEEDED  PartitionMemoryBudget=1024  PartitionMethod=ROBUST
  Tibia : sm_lib/Body Elements/File Solid  ExtGeomFileName=D:\Data\_PROGETTI\PRJ_SMART_SERVO\MATLAB\Arm Simulation\3D Models\tibia.stl  UnitType=Custom  ExtGeomFileUnits=mm  StepReaderType=HEX  ExportConvexHullGeometry=off  InertiaType=CalculateFromGeometry  Mass=1  MassUnits=kg  CenterOfMass=[0 0 0]  CenterOfMassUnits=m  MomentsOfInertia=[1 1 1]  MomentsOfInertiaUnits=kg*m^2  ProductsOfInertia=[0 0 0]  ProductsOfInertiaUnits=kg*m^2  BasedOnType=Density  Density=1200  DensityUnits=kg/m^3  DoExposeReferenceFrame=on  SerializedFrames=<Frames><Frame><Id>Frame1</Id><Value><Name>F1</Name><Origin><Source>ReferenceFrame</Source><FeatureName></FeatureName></Origin><PrimaryAxis><DefinedDirection>+Z</DefinedDirection><Source>ReferenceFrame</Source><SourceDirection>+Z</SourceDirection><FeatureName></FeatureName></PrimaryAxis><SecondaryAxis><DefinedDirection>+X</DefinedDirection><Source>ReferenceFrame</Source><SourceDirection>+X</SourceDirection><FeatureName></FeatureName></SecondaryAxis></Value></Frame></Frames>  GraphicType=FromGeometry  MarkerShape=Sphere  MarkerSize=10  GraphicVisPropType=SimpleVisualProperties  GraphicDiffuseColor=[1.0 0.2 0.2]  GraphicSpecularColor=[0.5 0.5 0.5 1.0]  GraphicAmbientColor=[0.15 0.15 0.15 1.0]  GraphicEmissiveColor=[0.0 0.0 0.0 1.0]  GraphicShininess=75  GraphicOpacity=1.0
  World Frame : sm_lib/Frames and Transforms/World Frame
  rotation : sm_lib/Frames and Transforms/Rigid Transform  TranslationMethod=None  TranslationStandardOffset=100  TranslationLengthUnit=mm  TranslationStandardAxis=+Z  TranslationCartesianOffset=[50 0 178]  TranslationROffset=0  TranslationROffsetUnits=m  TranslationZOffset=0  TranslationZOffsetUnits=m  TranslationThetaOffset=0  TranslationThetaOffsetUnits=deg  RotationMethod=StandardAxis  RotationAngleUnits=deg  RotationStandardAxis=+Z  RotationAngle=RotationAngle  RotationArbitraryAxis=[0 0 1]  FollAlignAxisA=+X  BaseAlignAxisA=+Y  FollAlignAxisB=+Y  BaseAlignAxisB=+Z  RotationSequenceAxes=FollowerAxes  RotationSequence=XYX  RotationSequenceAngles=[0 0 0]  RotationSequenceAnglesUnits=deg  RotationMatrix=[1 0 0; 0 1 0; 0 0 1]  Quaternion=[1 0 0 0]
  q1_m : Outport
  q2_m : Outport  Port=2
  q3_m : Outport  Port=3
  wires:
  PS-Simulink Converter/1 -> q1_m/1
  PS-Simulink Converter1/1 -> q2_m/1
  q_1/1 -> Simulink-PS Converter/1
  PS-Simulink Converter2/1 -> q3_m/1
  q_2/1 -> Simulink-PS Converter1/1
  q_3/1 -> Simulink-PS Converter2/1
  obstacle/1 -> Gain/1
  Gain/1 -> Simulink-PS Converter3/1
  connections:
  Simulink-PS Converter1/RConn1 -- Knee/LConn2
  Rigid Transform3/RConn1 -- Ankle/LConn1
  Ankle/RConn1 -- Tibia/LConn1
  Hip/RConn1 -- Rigid Transform2/LConn1 -- Coxa/LConn1
  Hip/LConn2 -- Simulink-PS Converter/RConn1
  Rigid Transform2/RConn1 -- Knee/LConn1
  Simulink-PS Converter2/RConn1 -- Ankle/LConn2
  Knee/RConn2 -- PS-Simulink Converter1/LConn1
  Hip/RConn2 -- PS-Simulink Converter/LConn1
  Knee/RConn1 -- Rigid Transform3/LConn1 -- Femur/RConn1
  Ankle/RConn2 -- PS-Simulink Converter2/LConn1
  Hip/LConn1 -- Rigid Transform1/RConn1
  Rigid Transform1/LConn1 -- rotation/RConn1
  Base/LConn1 -- Rigid Transform4/LConn1 -- Solver/RConn1 -- Configuration/RConn1 -- rotation/LConn1 -- World Frame/RConn1
  Simulink-PS Converter3/RConn1 -- Prismatic Joint/LConn2
  Prismatic Joint/RConn1 -- Obstacle/RConn1
  Prismatic Joint/LConn1 -- Rigid Transform4/RConn1

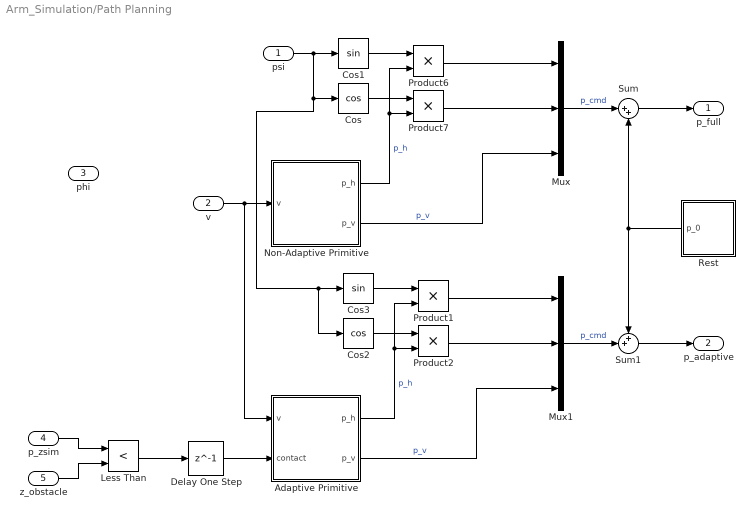
== system Arm_Simulation/Path Planning ==
  psi : Inport
  v : Inport  Port=2
  phi : Inport  Port=3
  p_zsim : Inport  Port=4
  z_obstacle : Inport  Port=5
  Adaptive Primitive : Subsystem  TreatAsAtomicUnit=on
  Cos : Trigonometry  Operator=cos
  Cos1 : Trigonometry
  Cos2 : Trigonometry  Operator=cos
  Cos3 : Trigonometry
  Delay One Step : Delay  DelayLength=1  SampleTime=1e-4
  Less Than : RelationalOperator  Operator=<  OutDataTypeStr=boolean  RndMeth=Simplest  InputSameDT=off
  Mux : Mux  Inputs=3
  Mux1 : Mux  Inputs=3
  Non-Adaptive Primitive : Subsystem  TreatAsAtomicUnit=on
  Product{1..2,6..7} (4 alike) : Product
  Rest : Subsystem
  Sum : Sum  Inputs=|++
  Sum1 : Sum  Inputs=++|
  p_full : Outport
  p_adaptive : Outport  Port=2
  wires:
  Sum/1 -> p_full/1
  Sum1/1 -> p_adaptive/1
  Rest/1(p_0) -> Sum1/1, Sum/2
  Mux/1 -> Sum/1  "p_cmd"
  v/1 -> Adaptive Primitive/1(v), Non-Adaptive Primitive/1(v)
  Non-Adaptive Primitive/1(p_h) -> Product7/2, Product6/2  "p_h"
  Non-Adaptive Primitive/2(p_v) -> Mux/3  "p_v"
  Cos/1 -> Product7/1
  Cos1/1 -> Product6/1
  Product6/1 -> Mux/1
  Product7/1 -> Mux/2
  p_zsim/1 -> Less Than/1
  z_obstacle/1 -> Less Than/2
  Less Than/1 -> Delay One Step/1
  Delay One Step/1 -> Adaptive Primitive/2(contact)
  Product2/1 -> Mux1/2
  Product1/1 -> Mux1/1
  psi/1 -> Cos3/1, Cos2/1, Cos/1, Cos1/1
  Cos3/1 -> Product1/1
  Cos2/1 -> Product2/1
  Adaptive Primitive/1(p_h) -> Product1/2, Product2/2  "p_h"
  Adaptive Primitive/2(p_v) -> Mux1/3  "p_v"
  Mux1/1 -> Sum1/2  "p_cmd"

== system Arm_Simulation/ Leg Geometric IK/CosineThrm 1 ==
  a : Inport
  b : Inport  Port=2
  c : Inport  Port=3
  Cos1 : Trigonometry  Operator=acos
  Divide : Product  Inputs=*/
  Gain : Gain  Gain=2
  Product : Product
  Square : Math  Operator=square
  Square1 : Math  Operator=square
  Square2 : Math  Operator=square
  Sum : Sum  Inputs=|++
  Sum3 : Sum  Inputs=|-+
  alpha : Outport
  wires:
  Product/1 -> Gain/1
  Square2/1 -> Sum/2
  Square1/1 -> Sum/1
  a/1 -> Square/1
  b/1 -> Square1/1, Product/1
  c/1 -> Square2/1, Product/2
  Sum/1 -> Sum3/2
  Square/1 -> Sum3/1
  Cos1/1 -> alpha/1
  Divide/1 -> Cos1/1
  Gain/1 -> Divide/2
  Sum3/1 -> Divide/1

== system Arm_Simulation/ Leg Geometric IK/CosineThrm 2 ==
  a : Inport
  b : Inport  Port=2
  c : Inport  Port=3
  Cos1 : Trigonometry  Operator=acos
  Divide : Product  Inputs=*/
  Gain : Gain  Gain=2
  Product : Product
  Square : Math  Operator=square
  Square1 : Math  Operator=square
  Square2 : Math  Operator=square
  Sum : Sum  Inputs=|++
  Sum3 : Sum  Inputs=|-+
  alpha : Outport
  wires:
  c/1 -> Product/2, Square2/1
  b/1 -> Product/1, Square1/1
  a/1 -> Square/1
  Square1/1 -> Sum/1
  Square2/1 -> Sum/2
  Product/1 -> Gain/1
  Sum/1 -> Sum3/2
  Square/1 -> Sum3/1
  Cos1/1 -> alpha/1
  Divide/1 -> Cos1/1
  Gain/1 -> Divide/2
  Sum3/1 -> Divide/1

== system Arm_Simulation/ Leg Geometric IK/Pythagora 1 ==
  c1 : Inport
  c2 : Inport  Port=2
  Sqrt : Sqrt
  Square : Math  Operator=square
  Square1 : Math  Operator=square
  Sum : Sum  Inputs=|++
  h : Outport
  wires:
  Sum/1 -> Sqrt/1
  c1/1 -> Square/1
  Square/1 -> Sum/1
  Square1/1 -> Sum/2
  c2/1 -> Square1/1
  Sqrt/1 -> h/1

== system Arm_Simulation/ Leg Geometric IK/Pythagora 2 ==
  c1 : Inport
  c2 : Inport  Port=2
  Sqrt : Sqrt
  Square : Math  Operator=square
  Square1 : Math  Operator=square
  Sum : Sum  Inputs=|++
  h : Outport
  wires:
  Sqrt/1 -> h/1
  c2/1 -> Square1/1
  Square1/1 -> Sum/2
  Square/1 -> Sum/1
  c1/1 -> Square/1
  Sum/1 -> Sqrt/1

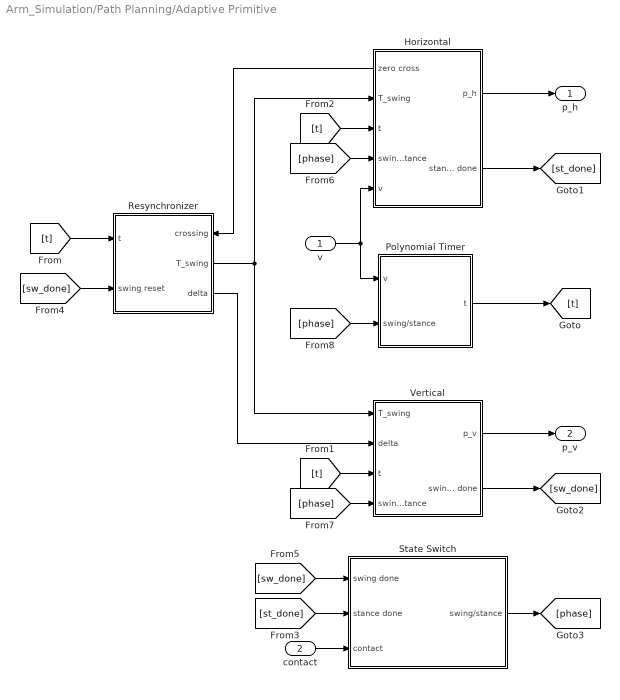
== system Arm_Simulation/Path Planning/Adaptive Primitive ==
  v : Inport
  contact : Inport  Port=2
  Horizontal : Subsystem
      settings: PortSchema="{\"entries\":[{\"content\":{\"sides\":[{\"content\":{\"connectorIds\":[\"Out3\",\"In1\",\"In2\",\"In3\",\"In4\"]},\"type\":\"ConnectorPlacement.EquallySpacedRectSide\",\"uuid\":\"130993a3-9dd7-498f-9637-003458af1e12\"},{\"content\":{\"connectorIds\":[\"Out1\",\"Out2\"],\"side\":\"RIGHT\"},\"type\":\"ConnectorPlacement.EquallySpacedRectSide\",\"uuid\":\"2f31e0ef-3848-4b5d-858d-873934ce2c21\"},{\"content\":{\"connectorIds\":[],\"side\":\"TOP\"},\"type\":\"ConnectorPlacement.EquallySpacedRectSide\",\"uuid\":\"f8541dc5-0eca-42df-927e-cf9786e19294\"}]},\"type\":\"ConnectorPlacement.EquallySpacedConnector\",\"uuid\":\"a2deafe6-24bc-411c-9ec2-6aaa7e72c1e2\"}],\"packageUris\":[\"http://schema.mathworks.com/mf0/Connector/R2020b\"],\"version\":\"1.0\"}"
  Polynomial Timer : Subsystem
  Resynchronizer : Subsystem
      settings: PortSchema="{\"entries\":[{\"content\":{\"sides\":[{\"content\":{\"connectorIds\":[\"In1\",\"In2\"]},\"type\":\"ConnectorPlacement.EquallySpacedRectSide\",\"uuid\":\"62c16c4d-254c-4f19-ac82-c5564fd87460\"},{\"content\":{\"connectorIds\":[\"In3\",\"Out1\",\"Out2\"],\"side\":\"RIGHT\"},\"type\":\"ConnectorPlacement.EquallySpacedRectSide\",\"uuid\":\"75ae3a29-aa01-4e70-aab2-f18b5b67135b\"},{\"content\":{\"connectorIds\":[],\"side\":\"TOP\"},\"type\":\"ConnectorPlacement.EquallySpacedRectSide\",\"uuid\":\"8528bca1-e229-43e3-9560-3c949121943b\"},{\"content\":{\"connectorIds\":[],\"side\":\"BOTTOM\"},\"type\":\"ConnectorPlacement.EquallySpacedRectSide\",\"uuid\":\"2e3eb36b-ba67-4841-99ba-214bcdf47ea9\"}]},\"type\":\"ConnectorPlacement.EquallySpacedConnector\",\"uuid\":\"92c07b80-2243-4296-a92d-df0c5d1b7140\"}],\"packageUris\":[\"http://schema.mathworks.com/mf0/Connector/R2020b\"],\"version\":\"1.0\"}"
  State Switch : Subsystem
      settings: PortSchema="{\"entries\":[{\"content\":{\"sides\":[{\"content\":{\"connectorIds\":[\"Out1\"]},\"type\":\"ConnectorPlacement.EquallySpacedRectSide\",\"uuid\":\"6334b3b7-75d3-4d81-afc4-23195bb8d279\"},{\"content\":{\"connectorIds\":[\"In1\",\"In2\",\"In3\"],\"side\":\"RIGHT\"},\"type\":\"ConnectorPlacement.EquallySpacedRectSide\",\"uuid\":\"708193af-67b3-42bc-9844-21b807bd9e01\"},{\"content\":{\"connectorIds\":[],\"side\":\"TOP\"},\"type\":\"ConnectorPlacement.EquallySpacedRectSide\",\"uuid\":\"afc6b7d0-f1e8-4474-802e-26aa198a325f\"}]},\"type\":\"ConnectorPlacement.EquallySpacedConnector\",\"uuid\":\"983320bd-7b6c-49a1-9b2d-1e02992f6dfe\"}],\"packageUris\":[\"http://schema.mathworks.com/mf0/Connector/R2020b\"],\"version\":\"1.0\"}"
  Vertical : Subsystem
  p_h : Outport
  p_v : Outport  Port=2
  wires:
  v/1 -> Polynomial Timer/1(v), Horizontal/4(v)
  Horizontal/1(p_h) -> p_h/1
  Vertical/1(p_v) -> p_v/1
  [sw_done] -> State Switch/1(swing done)
  contact/1 -> State Switch/3(contact)
  Horizontal/3(zero cross) -> Resynchronizer/3(crossing)
  Resynchronizer/2(delta) -> Vertical/2(delta)
  Resynchronizer/1(T_swing) -> Horizontal/1(T_swing), Vertical/1(T_swing)
  Polynomial Timer/1(t) -> [t]
  [t] -> Resynchronizer/1(t)
  [t] -> Vertical/3(t)
  [t] -> Horizontal/2(t)
  Horizontal/2(stance done) -> [st_done]
  [st_done] -> State Switch/2(stance done)
  Vertical/2(swing done) -> [sw_done]
  [sw_done] -> Resynchronizer/2(swing reset)
  State Switch/1(swing/stance) -> [phase]
  [phase] -> Horizontal/3(swing/stance)
  [phase] -> Vertical/4(swing/stance)
  [phase] -> Polynomial Timer/2(swing/stance)

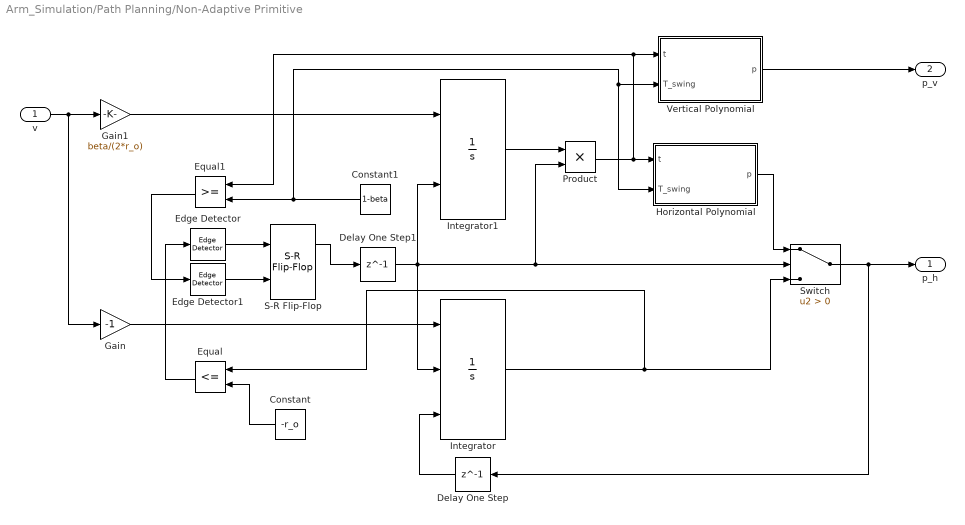
== system Arm_Simulation/Path Planning/Non-Adaptive Primitive ==
  v : Inport
  Constant : Constant  Value=-r_o
  Constant1 : Constant  Value=1-beta
  Delay One Step : Delay  DelayLength=1  SampleTime=1e-4
  Delay One Step1 : Delay  DelayLength=1  SampleTime=1e-4
  Edge Detector : spsEdgeDetectorLib/Edge Detector  model=Rising  ic=0  Ts=1e-4
      settings: LibrarySourceBlock=sps_lib/Control/Edge Detector
  Edge Detector1 : spsEdgeDetectorLib/Edge Detector  model=Rising  ic=0  Ts=1e-4
      settings: LibrarySourceBlock=sps_lib/Control/Edge Detector
  Equal : RelationalOperator  Operator=<=  OutDataTypeStr=boolean  RndMeth=Simplest  InputSameDT=off
  Equal1 : RelationalOperator  OutDataTypeStr=boolean  RndMeth=Simplest  InputSameDT=off
  Gain : Gain  Gain=-1
  Gain1 : Gain  Gain=beta/(2*r_o)
  Horizontal Polynomial : MATLAB Function  TreatAsAtomicUnit=on
  Integrator : Integrator  ExternalReset=falling  InitialConditionSource=external
  Integrator1 : Integrator  ExternalReset=rising
  Product : Product
  S-R Flip-Flop : simulink_extras/Flip Flops/S-R Flip-Flop  initial_condition=0
  Switch : Switch  Criteria=u2 > Threshold  SaturateOnIntegerOverflow=off  InputSameDT=off
  Vertical Polynomial : MATLAB Function  TreatAsAtomicUnit=on
  p_h : Outport
  p_v : Outport  Port=2
  wires:
  Gain/1 -> Integrator/1
  v/1 -> Gain/1, Gain1/1
  Product/1 -> Equal1/1, Vertical Polynomial/1(t), Horizontal Polynomial/1(t)
  Gain1/1 -> Integrator1/1
  Switch/1 -> p_h/1, Delay One Step/1
  Delay One Step/1 -> Integrator/3
  Horizontal Polynomial/1(p) -> Switch/1
  Constant/1 -> Equal/2
  Constant1/1 -> Horizontal Polynomial/2(T_swing), Vertical Polynomial/2(T_swing), Equal1/2
  Equal1/1 -> Edge Detector1/1
  Equal/1 -> Edge Detector/1
  S-R Flip-Flop/1 -> Delay One Step1/1
  Integrator/1 -> Switch/3, Equal/1
  Edge Detector/1 -> S-R Flip-Flop/1
  Edge Detector1/1 -> S-R Flip-Flop/2
  Vertical Polynomial/1(p) -> p_v/1
  Integrator1/1 -> Product/1
  Delay One Step1/1 -> Product/2, Switch/2, Integrator/2, Integrator1/2

== system Arm_Simulation/Path Planning/Rest ==
  Constant2 : Constant  Value=Cx
  Constant3 : Constant  Value=Cy
  Constant4 : Constant  Value=Cz
  Mux1 : Mux  Inputs=3
  p_0 : Outport
  wires:
  Constant4/1 -> Mux1/3  "p_0z"
  Constant3/1 -> Mux1/2  "p_0y"
  Constant2/1 -> Mux1/1  "p_0x"
  Mux1/1 -> p_0/1  "p_0"

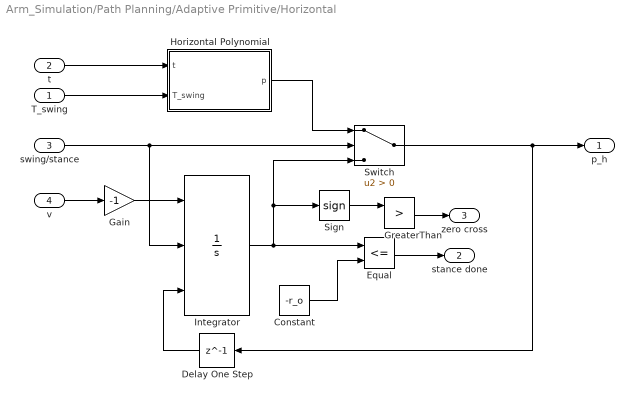
== system Arm_Simulation/Path Planning/Adaptive Primitive/Horizontal ==
  T_swing : Inport
  t : Inport  Port=2
  swing/stance : Inport  Port=3
  v : Inport  Port=4
  Constant : Constant  Value=-r_o
  Delay One Step : Delay  DelayLength=1  SampleTime=1e-4
  Equal : RelationalOperator  Operator=<=  OutDataTypeStr=boolean  RndMeth=Simplest  InputSameDT=off
  Gain : Gain  Gain=-1
  GreaterThan : RelationalOperator  Operator=>  OutDataTypeStr=boolean  RndMeth=Simplest  InputSameDT=off
  Horizontal Polynomial : MATLAB Function  TreatAsAtomicUnit=on
  Integrator : Integrator  ExternalReset=falling  InitialConditionSource=external
  Sign : Signum
  Switch : Switch  Criteria=u2 > Threshold  SaturateOnIntegerOverflow=off  InputSameDT=off
  p_h : Outport
  stance done : Outport  Port=2
  zero cross : Outport  Port=3
  wires:
  Switch/1 -> p_h/1, Delay One Step/1
  Constant/1 -> Equal/2
  Delay One Step/1 -> Integrator/3
  Gain/1 -> Integrator/1
  T_swing/1 -> Horizontal Polynomial/2(T_swing)
  Horizontal Polynomial/1(p) -> Switch/1
  Equal/1 -> stance done/1
  t/1 -> Horizontal Polynomial/1(t)
  v/1 -> Gain/1
  swing/stance/1 -> Switch/2, Integrator/2
  Sign/1 -> GreaterThan/1
  Integrator/1 -> Sign/1, Switch/3, Equal/1
  GreaterThan/1 -> zero cross/1

== system Arm_Simulation/Path Planning/Adaptive Primitive/Polynomial Timer ==
  v : Inport
  swing/stance : Inport  Port=2
  Gain1 : Gain  Gain=beta/(2*r_o)
  Integrator1 : Integrator  ExternalReset=rising
  t : Outport
  wires:
  Gain1/1 -> Integrator1/1
  v/1 -> Gain1/1
  swing/stance/1 -> Integrator1/2
  Integrator1/1 -> t/1

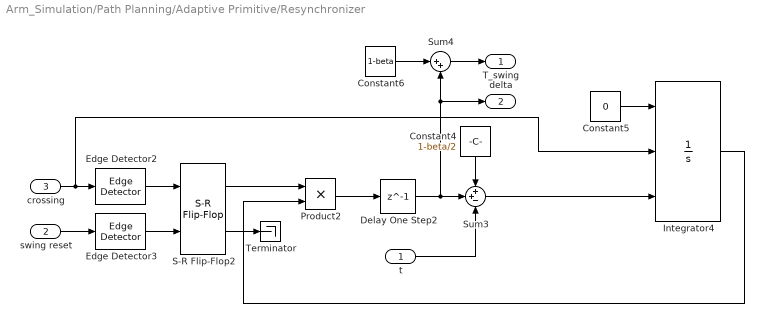
== system Arm_Simulation/Path Planning/Adaptive Primitive/Resynchronizer ==
  t : Inport
  swing reset : Inport  Port=2
  crossing : Inport  Port=3
  Constant4 : Constant  Value=1-beta/2
  Constant5 : Constant  Value=0
  Constant6 : Constant  Value=1-beta
  Delay One Step2 : Delay  DelayLength=1  SampleTime=1e-4
  Edge Detector2 : spsEdgeDetectorLib/Edge Detector  model=Falling  ic=0  Ts=1e-4
      settings: LibrarySourceBlock=sps_lib/Control/Edge Detector
  Edge Detector3 : spsEdgeDetectorLib/Edge Detector  model=Falling  ic=0  Ts=1e-4
      settings: LibrarySourceBlock=sps_lib/Control/Edge Detector
  Integrator4 : Integrator  ExternalReset=falling  InitialConditionSource=external
  Product2 : Product
  S-R Flip-Flop2 : simulink_extras/Flip Flops/S-R Flip-Flop  initial_condition=0
  Sum3 : Sum  Inputs=++-
  Sum4 : Sum  Inputs=|++
  Terminator : Terminator
  T_swing : Outport
  delta : Outport  Port=2
  wires:
  Sum4/1 -> T_swing/1
  Sum3/1 -> Integrator4/3
  S-R Flip-Flop2/1 -> Product2/1
  Edge Detector2/1 -> S-R Flip-Flop2/1
  crossing/1 -> Edge Detector2/1, Integrator4/2
  Constant4/1 -> Sum3/1
  Edge Detector3/1 -> S-R Flip-Flop2/2
  Integrator4/1 -> Product2/2
  Constant5/1 -> Integrator4/1
  S-R Flip-Flop2/2 -> Terminator/1
  Constant6/1 -> Sum4/1
  swing reset/1 -> Edge Detector3/1
  t/1 -> Sum3/3
  Product2/1 -> Delay One Step2/1
  Delay One Step2/1 -> delta/1, Sum4/2, Sum3/2

== system Arm_Simulation/Path Planning/Adaptive Primitive/State Switch ==
  swing done : Inport
  stance done : Inport  Port=2
  contact : Inport  Port=3
  Delay One Step1 : Delay  DelayLength=1  SampleTime=1e-4
  Edge Detector : spsEdgeDetectorLib/Edge Detector  model=Rising  ic=0  Ts=1e-4
      settings: LibrarySourceBlock=sps_lib/Control/Edge Detector
  Edge Detector2 : spsEdgeDetectorLib/Edge Detector  model=Rising  ic=0  Ts=1e-4
      settings: LibrarySourceBlock=sps_lib/Control/Edge Detector
  OR : Logic  Operator=OR  IconShape=distinctive  AllPortsSameDT=off  OutDataTypeStr=boolean
  S-R Flip-Flop1 : simulink_extras/Flip Flops/S-R Flip-Flop  initial_condition=0
  Terminator1 : Terminator
  swing/stance : Outport
  wires:
  S-R Flip-Flop1/1 -> Delay One Step1/1
  stance done/1 -> Edge Detector/1
  OR/1 -> Edge Detector2/1
  contact/1 -> OR/2
  Edge Detector/1 -> S-R Flip-Flop1/1
  swing done/1 -> OR/1
  Edge Detector2/1 -> S-R Flip-Flop1/2
  Delay One Step1/1 -> swing/stance/1
  S-R Flip-Flop1/2 -> Terminator1/1

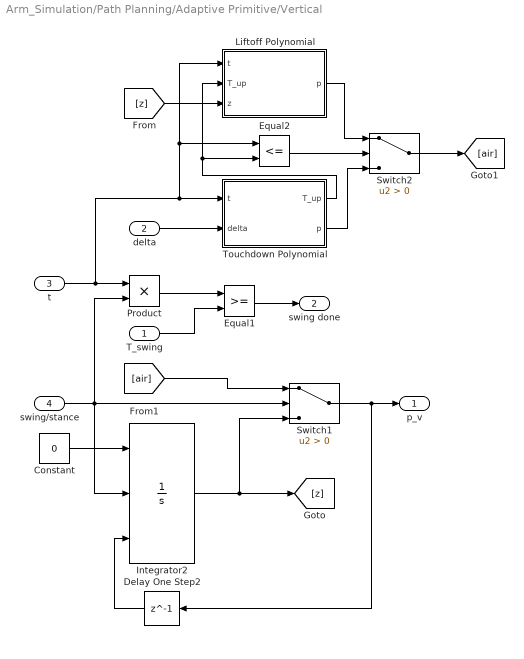
== system Arm_Simulation/Path Planning/Adaptive Primitive/Vertical ==
  T_swing : Inport
  delta : Inport  Port=2
  t : Inport  Port=3
  swing/stance : Inport  Port=4
  Constant : Constant  Value=0
  Delay One Step2 : Delay  DelayLength=1  SampleTime=1e-4
  Equal1 : RelationalOperator  OutDataTypeStr=boolean  RndMeth=Simplest  InputSameDT=off
  Equal2 : RelationalOperator  Operator=<=  OutDataTypeStr=boolean  RndMeth=Simplest  InputSameDT=off
  Integrator2 : Integrator  ExternalReset=falling  InitialConditionSource=external
  Liftoff Polynomial : MATLAB Function  TreatAsAtomicUnit=on
  Product : Product
  Switch1 : Switch  Criteria=u2 > Threshold  SaturateOnIntegerOverflow=off  InputSameDT=off
  Switch2 : Switch  Criteria=u2 > Threshold  SaturateOnIntegerOverflow=off  InputSameDT=off
  Touchdown Polynomial : MATLAB Function  TreatAsAtomicUnit=on
  p_v : Outport
  swing done : Outport  Port=2
  wires:
  Equal1/1 -> swing done/1
  Switch1/1 -> p_v/1, Delay One Step2/1
  Delay One Step2/1 -> Integrator2/3
  Integrator2/1 -> [z], Switch1/3
  Constant/1 -> Integrator2/1
  Touchdown Polynomial/2(p) -> Switch2/3
  Liftoff Polynomial/1(p) -> Switch2/1
  Equal2/1 -> Switch2/2
  Switch2/1 -> [air]
  delta/1 -> Touchdown Polynomial/2(delta)
  swing/stance/1 -> Switch1/2, Product/2, Integrator2/2
  Product/1 -> Equal1/1
  [z] -> Liftoff Polynomial/3(z)
  T_swing/1 -> Equal1/2
  Touchdown Polynomial/1(T_up) -> Equal2/2, Liftoff Polynomial/2(T_up)
  [air] -> Switch1/1
  t/1 -> Product/1, Liftoff Polynomial/1(t), Equal2/1, Touchdown Polynomial/1(t)
